simulink model "isorc2016_1"  (Simulink 8.1)
settings: Solver=ode45  StartTime=0.0  StopTime=10.0  RelTol=1e-3
settings Model: Creator=fernando  LastModifiedBy=fernando
settings DataIOCC: SignalLoggingSaveFormat=Dataset
settings OptimizationCC: ExpressionDepthLimit=128
settings DebuggingCC: FcnCallInpInsideContextMsg=EnableAllAsError
settings GRTTargetCC: CombineOutputUpdateFcns=on  GRTInterface=off

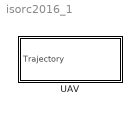
== system isorc2016_1 ==
  UAV : Subsystem  RequirementInfo="{}  %GIDa_5af21c82_02ae_4032_b775_208782874602"
      settings: AttributesFormatString=system

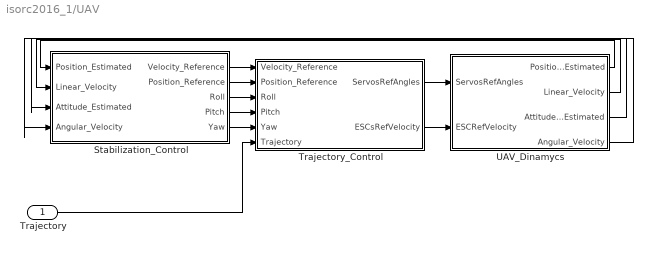
== system isorc2016_1/UAV ==
  Trajectory : Inport
  Stabilization_Control : Subsystem
      settings: AttributesFormatString=process/thread
  Trajectory_Control : Subsystem
      settings: AttributesFormatString=process/thread
  UAV_Dinamycs : Subsystem
      settings: AttributesFormatString=device
  wires:
  UAV_Dinamycs/1(Position_Estimated) -> Stabilization_Control/1(Position_Estimated)
  UAV_Dinamycs/3(Attitude_Estimated) -> Stabilization_Control/3(Attitude_Estimated)
  UAV_Dinamycs/2(Linear_Velocity) -> Stabilization_Control/2(Linear_Velocity)
  UAV_Dinamycs/4(Angular_Velocity) -> Stabilization_Control/4(Angular_Velocity)
  Stabilization_Control/5(Yaw) -> Trajectory_Control/5(Yaw)
  Stabilization_Control/4(Pitch) -> Trajectory_Control/4(Pitch)
  Stabilization_Control/2(Position_Reference) -> Trajectory_Control/2(Position_Reference)
  Stabilization_Control/3(Roll) -> Trajectory_Control/3(Roll)
  Stabilization_Control/1(Velocity_Reference) -> Trajectory_Control/1(Velocity_Reference)
  Trajectory_Control/1(ServosRefAngles) -> UAV_Dinamycs/1(ServosRefAngles)
  Trajectory_Control/2(ESCsRefVelocity) -> UAV_Dinamycs/2(ESCRefVelocity)
  Trajectory/1 -> Trajectory_Control/6(Trajectory)

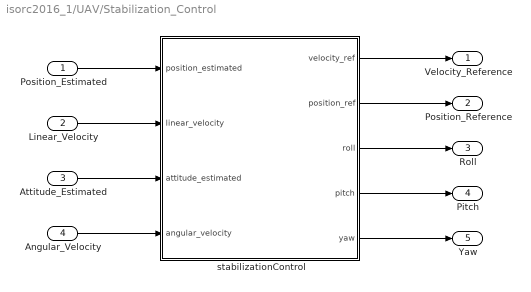
== system isorc2016_1/UAV/Stabilization_Control ==
  Position_Estimated : Inport
  Linear_Velocity : Inport  Port=2
  Attitude_Estimated : Inport  Port=3
  Angular_Velocity : Inport  Port=4
  stabilizationControl : MATLAB Function  TreatAsAtomicUnit=on
  Velocity_Reference : Outport
  Position_Reference : Outport  Port=2
  Roll : Outport  Port=3
  Pitch : Outport  Port=4
  Yaw : Outport  Port=5
  wires:
  Linear_Velocity/1 -> stabilizationControl/2(linear_velocity)
  Position_Estimated/1 -> stabilizationControl/1(position_estimated)
  Angular_Velocity/1 -> stabilizationControl/4(angular_velocity)
  Attitude_Estimated/1 -> stabilizationControl/3(attitude_estimated)
  stabilizationControl/1(velocity_ref) -> Velocity_Reference/1
  stabilizationControl/2(position_ref) -> Position_Reference/1
  stabilizationControl/3(roll) -> Roll/1
  stabilizationControl/4(pitch) -> Pitch/1
  stabilizationControl/5(yaw) -> Yaw/1

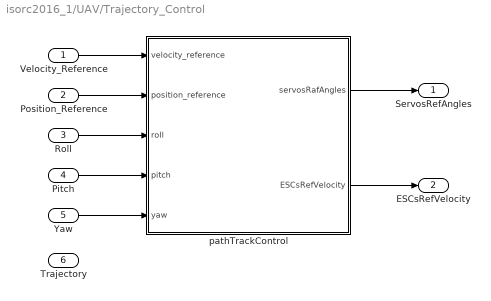
== system isorc2016_1/UAV/Trajectory_Control ==
  Velocity_Reference : Inport
  Position_Reference : Inport  Port=2
  Roll : Inport  Port=3
  Pitch : Inport  Port=4
  Yaw : Inport  Port=5
  Trajectory : Inport  Port=6
  pathTrackControl : MATLAB Function  TreatAsAtomicUnit=on
  ServosRefAngles : Outport
  ESCsRefVelocity : Outport  Port=2
  wires:
  Pitch/1 -> pathTrackControl/4(pitch)
  Roll/1 -> pathTrackControl/3(roll)
  Position_Reference/1 -> pathTrackControl/2(position_reference)
  Yaw/1 -> pathTrackControl/5(yaw)
  Velocity_Reference/1 -> pathTrackControl/1(velocity_reference)
  pathTrackControl/1(servosRafAngles) -> ServosRefAngles/1
  pathTrackControl/2(ESCsRefVelocity) -> ESCsRefVelocity/1

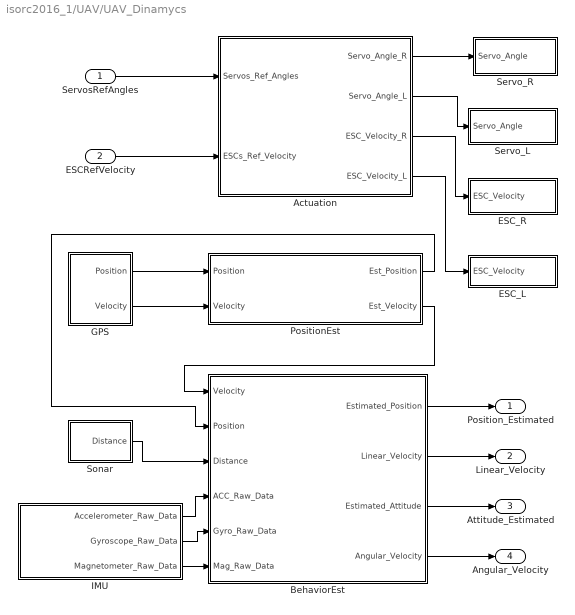
== system isorc2016_1/UAV/UAV_Dinamycs ==
  ServosRefAngles : Inport
  ESCRefVelocity : Inport  Port=2
  Actuation : Subsystem
      settings: AttributesFormatString=thread
  BehaviorEst : Subsystem
      settings: AttributesFormatString=thread
  ESC_L : Subsystem
      settings: AttributesFormatString=device
  ESC_R : Subsystem
      settings: AttributesFormatString=device
  GPS : Subsystem
      settings: AttributesFormatString=device
  IMU : Subsystem
      settings: AttributesFormatString=device
  PositionEst : Subsystem
      settings: AttributesFormatString=thread
  Servo_L : Subsystem
      settings: AttributesFormatString=device
  Servo_R : Subsystem
      settings: AttributesFormatString=device
  Sonar : Subsystem
      settings: AttributesFormatString=device
  Position_Estimated : Outport
  Linear_Velocity : Outport  Port=2
  Attitude_Estimated : Outport  Port=3
  Angular_Velocity : Outport  Port=4
  wires:
  ServosRefAngles/1 -> Actuation/1(Servos_Ref_Angles)
  ESCRefVelocity/1 -> Actuation/2(ESCs_Ref_Velocity)
  Actuation/1(Servo_Angle_R) -> Servo_R/1(Servo_Angle)
  Actuation/2(Servo_Angle_L) -> Servo_L/1(Servo_Angle)
  Actuation/3(ESC_Velocity_R) -> ESC_R/1(ESC_Velocity)
  Actuation/4(ESC_Velocity_L) -> ESC_L/1(ESC_Velocity)
  GPS/1(Position) -> PositionEst/1(Position)
  GPS/2(Velocity) -> PositionEst/2(Velocity)
  Sonar/1(Distance) -> BehaviorEst/3(Distance)
  IMU/1(Accelerometer_Raw_Data) -> BehaviorEst/4(ACC_Raw_Data)
  IMU/2(Gyroscope_Raw_Data) -> BehaviorEst/5(Gyro_Raw_Data)
  IMU/3(Magnetometer_Raw_Data) -> BehaviorEst/6(Mag_Raw_Data)
  PositionEst/1(Est_Position) -> BehaviorEst/2(Position)
  PositionEst/2(Est_Velocity) -> BehaviorEst/1(Velocity)
  BehaviorEst/1(Estimated_Position) -> Position_Estimated/1
  BehaviorEst/2(Linear_Velocity) -> Linear_Velocity/1
  BehaviorEst/3(Estimated_Attitude) -> Attitude_Estimated/1
  BehaviorEst/4(Angular_Velocity) -> Angular_Velocity/1

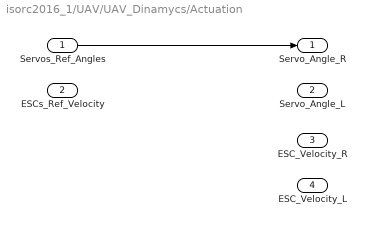
== system isorc2016_1/UAV/UAV_Dinamycs/Actuation ==
  Servos_Ref_Angles : Inport
  ESCs_Ref_Velocity : Inport  Port=2
  Servo_Angle_R : Outport
  Servo_Angle_L : Outport  Port=2
  ESC_Velocity_R : Outport  Port=3
  ESC_Velocity_L : Outport  Port=4
  wires:
  Servos_Ref_Angles/1 -> Servo_Angle_R/1

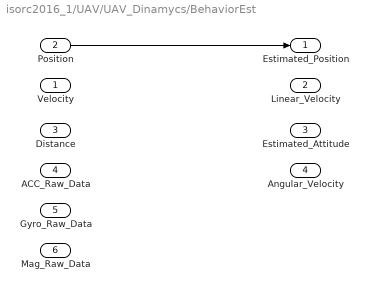
== system isorc2016_1/UAV/UAV_Dinamycs/BehaviorEst ==
  Velocity : Inport
  Position : Inport  Port=2
  Distance : Inport  Port=3
  ACC_Raw_Data : Inport  Port=4
  Gyro_Raw_Data : Inport  Port=5
  Mag_Raw_Data : Inport  Port=6
  Estimated_Position : Outport
  Linear_Velocity : Outport  Port=2
  Estimated_Attitude : Outport  Port=3
  Angular_Velocity : Outport  Port=4
  wires:
  Position/1 -> Estimated_Position/1

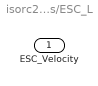
== system isorc2016_1/UAV/UAV_Dinamycs/ESC_L ==
  ESC_Velocity : Inport

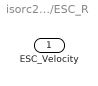
== system isorc2016_1/UAV/UAV_Dinamycs/ESC_R ==
  ESC_Velocity : Inport

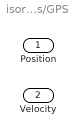
== system isorc2016_1/UAV/UAV_Dinamycs/GPS ==
  Position : Outport
  Velocity : Outport  Port=2

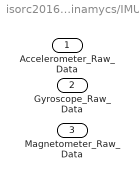
== system isorc2016_1/UAV/UAV_Dinamycs/IMU ==
  Accelerometer_Raw_Data : Outport
  Gyroscope_Raw_Data : Outport  Port=2
  Magnetometer_Raw_Data : Outport  Port=3

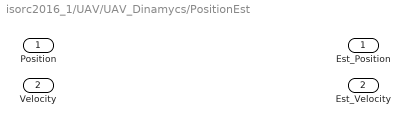
== system isorc2016_1/UAV/UAV_Dinamycs/PositionEst ==
  Position : Inport
  Velocity : Inport  Port=2
  Est_Position : Outport
  Est_Velocity : Outport  Port=2

== system isorc2016_1/UAV/UAV_Dinamycs/Servo_L ==
  Servo_Angle : Inport

== system isorc2016_1/UAV/UAV_Dinamycs/Servo_R ==
  Servo_Angle : Inport

== system isorc2016_1/UAV/UAV_Dinamycs/Sonar ==
  Distance : Outport

== matlab function UAV/Trajectory_Control/pathTrackControl ==
  data: velocity_reference input double; servosRafAngles output double; position_reference input double; roll input double; pitch input double; yaw input double; ESCsRefVelocity output double
function [servosRafAngles,ESCsRefVelocity]= pathTrack(velocity_reference, position_reference,roll, pitch,yaw)
%#codegen

y = u;

== matlab function UAV/Stabilization_Control/stabilizationControl ==
  data: position_estimated input double; velocity_ref output double; linear_velocity input double; attitude_estimated input double; angular_velocity input double; position_ref output double; roll output double; pitch output double; yaw output double
function [velocity_ref,position_ref,roll,pitch,yaw]= stabilizationControl(position_estimated,linear_velocity,attitude_estimated,angular_velocity)
%#codegen

y = u;
